simulink model "cuatro_cuadr_model"  (R2018b)
settings: Solver=VariableStepAuto  StartTime=0.0  StopTime=50  RelTol=1e-3
PreLoadFcn:
  | model_parameters.m
values from neighbouring files (symbols this model uses):
  ba = Jeq * wv    (= 1.911)    [cuatro_cuadr_const.m]
  beq = 0.01    [cuatro_cuadr_const.m]
  Jeq = 0.026    [cuatro_cuadr_const.m]
  Ke = 1.795    [cuatro_cuadr_const.m]
  kisa = ksa * wi    (= 240.786)    [cuatro_cuadr_const.m]
  ksa = ba * wpos    (= 40.131)    [cuatro_cuadr_const.m]
  Kt = 1.795    [cuatro_cuadr_const.m]
  La = 40.5e-3    (= 0.0405)    [cuatro_cuadr_const.m]
  Le = 44    [cuatro_cuadr_const.m]
  P = 2.2e3    (= 2200)    [cuatro_cuadr_const.m]
  Ra = 10.7    [cuatro_cuadr_const.m]
  Re = 220    [cuatro_cuadr_const.m]
  Tau = 0.001    [crane_constants.m]    (also in cuatro_cuadr_const.m)
libraries: simulink x1
settings Model: Creator=jere  LastModifiedBy=Jere
settings DebuggingCC: LibraryContextMissingDiagnostic=none
settings SFSimCC: SimUseLocalCustomCode=off
settings RTWCC: RTWUseLocalCustomCode=off

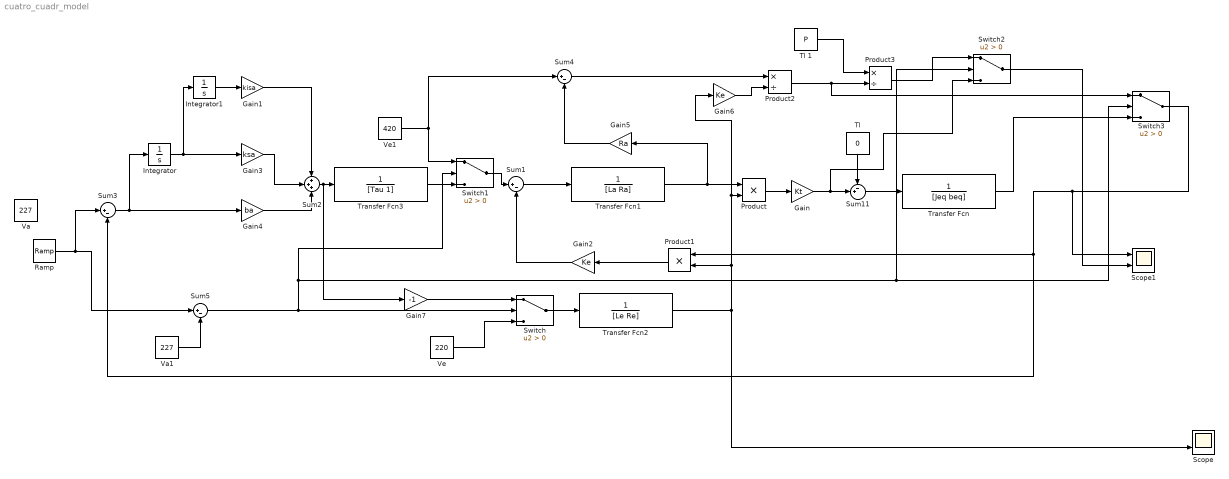
== system cuatro_cuadr_model ==
  Gain : Gain  Gain=Kt
  Gain1 : Gain  Gain=kisa
  Gain2 : Gain  Gain=Ke
  Gain3 : Gain  Gain=ksa
  Gain4 : Gain  Gain=ba
  Gain5 : Gain  Gain=Ra
  Gain6 : Gain  Gain=Ke
  Gain7 : Gain  Gain=-1
  Integrator : Integrator
  Integrator1 : Integrator
  Product : Product
  Product1 : Product
  Product2 : Product  Inputs=*/
  Product3 : Product  Inputs=*/
  Ramp : simulink/Sources/Ramp  slope=10  start=0  InitialOutput=0
  Scope : Scope  NumInputPorts=2
  Scope1 : Scope  NumInputPorts=2
  Sum{1,3..5} (4 alike) : Sum  Inputs=|+-
  Sum11 : Sum  Inputs=-+|
  Sum2 : Sum  Inputs=+++
  Switch{,1..3} (4 alike) : Switch  Criteria=u2 > Threshold
  "Tl " : Constant  Value=0
  Tl 1 : Constant  Value=P
  Transfer Fcn : TransferFcn  Denominator=[Jeq beq]
  Transfer Fcn1 : TransferFcn  Denominator=[La Ra]
  Transfer Fcn2 : TransferFcn  Denominator=[Le Re]
  Transfer Fcn3 : TransferFcn  Denominator=[Tau 1]
  Va : Constant  Value=227
  Va1 : Constant  Value=227
  Ve : Constant  Value=220
  Ve1 : Constant  Value=420
  wires:
  Sum11/1 -> Transfer Fcn/1
  "Tl "/1 -> Sum11/1
  Gain/1 -> Switch2/3, Sum11/2
  Transfer Fcn1/1 -> Gain5/1, Product/1
  Product/1 -> Gain/1
  Transfer Fcn2/1 -> Gain6/1, Product/2, Product1/2, Scope/2
  Sum1/1 -> Transfer Fcn1/1
  Product1/1 -> Gain2/1
  Gain2/1 -> Sum1/2
  Switch3/1 -> Sum3/2, Product1/1, Scope1/1
  Sum2/1 -> Gain7/1, Transfer Fcn3/1
  Sum3/1 -> Integrator/1, Gain4/1
  Gain1/1 -> Sum2/1
  Gain3/1 -> Sum2/2
  Gain4/1 -> Sum2/3
  Integrator/1 -> Integrator1/1, Gain3/1
  Integrator1/1 -> Gain1/1
  Ve1/1 -> Switch1/1, Sum4/1
  Gain5/1 -> Sum4/2
  Sum4/1 -> Product2/1
  Gain6/1 -> Product2/2
  Product2/1 -> Switch3/1, Product3/2
  Tl 1/1 -> Product3/1
  Transfer Fcn3/1 -> Switch1/3
  Switch1/1 -> Sum1/1
  Ve/1 -> Switch/3
  Switch/1 -> Transfer Fcn2/1
  Product3/1 -> Switch2/1
  Switch2/1 -> Scope1/2
  Transfer Fcn/1 -> Switch3/3
  Gain7/1 -> Switch/1
  Va1/1 -> Sum5/2
  Sum5/1 -> Switch3/2, Switch2/2, Switch1/2, Switch/2
  Ramp/1 -> Sum5/1, Sum3/1
